simulink model "ANS_GFM_short_term"  (R2021b)
settings: Solver=FixedStepAuto  StartTime=0.0  StopTime=5  FixedStep=Ts  MaxStep=1e-5  RelTol=1e-3
values from neighbouring files (symbols this model uses):
  angle_load = angle(LF.bus(ind_l).Vbus)*180/pi    [init_ANS_GFM_long_term.m]    (also in init_ANS_GFM_short_term.m)
  angleV_LF = Vangle_init/180*pi    [init_ANS_GFM_long_term.m]    (also in init_ANS_GFM_short_term.m)
  awu = 1    [init_ANS_GFM_long_term.m]    (also in init_ANS_GFM_short_term.m)
  C_dc = 1/(Xcdc_pu_or*Zbase_dc_new*100*pi)    [init_ANS_GFM_long_term.m]    (also in init_ANS_GFM_short_term.m)
  C_f = 1/(Xcf_pu_or*Zbase_new*100*pi)    (= 0.013712)    [init_ANS_GFM_long_term.m]    (also in init_ANS_GFM_short_term.m = 0.0141333333333)
  control = 3    [init_ANS_GFM_long_term.m]    (also in init_ANS_GFM_short_term.m = 1)
  D_p = (1/(m_p*w_b))    (= 5209935.26289)    [init_ANS_GFM_long_term.m]    (also in init_ANS_GFM_short_term.m = 5370022.73304)
  Egrid_tmp = 1.054080675694902*400e3    (= 421632.270278)    [init_ANS_GFM_long_term.m]    (also in init_ANS_GFM_short_term.m)
  epsi = 1e-4    (= 0.0001)    [init_ANS_GFM_long_term.m]    (also in init_ANS_GFM_short_term.m)
  eta = m_p*V_m^2    [init_ANS_GFM_long_term.m]    (also in init_ANS_GFM_short_term.m)
  gamma = 2.3    [init_ANS_GFM_long_term.m]    (also in init_ANS_GFM_short_term.m)
  I0_init = [I0_init_a, I0_init_b, I0_init_c]    [init_ANS_GFM_long_term.m]    (also in init_ANS_GFM_short_term.m)
  I_bc = S_bc / (V_bc*sqrt(3))    [init_ANS_GFM_long_term.m]    (also in init_ANS_GFM_short_term.m)
  I_d_int_init = (U_d_int + I_q_int*L_f*w_b - V_d_int - I_d_int*R_f*0)    [init_ANS_GFM_long_term.m]    (also in init_ANS_GFM_short_term.m)
  I_init = [I_init_a, I_init_b, I_init_c]    [init_ANS_GFM_long_term.m]    (also in init_ANS_GFM_short_term.m)
  i_ll = -1.15*(S_bc/Vdc_n)-i_loss_dc    [init_ANS_GFM_long_term.m]    (also in init_ANS_GFM_short_term.m)
  I_max_sat_pu = 1.0 * I_bc *sqrt(2)    [init_ANS_GFM_long_term.m]    (also in init_ANS_GFM_short_term.m)
  I_q_int_init = (U_q_int - I_d_int*L_f*w_b - V_q_int - I_q_int*R_f*0)    [init_ANS_GFM_long_term.m]    (also in init_ANS_GFM_short_term.m)
  i_ul = 1.15*(S_bc/Vdc_n)+i_loss_dc    [init_ANS_GFM_long_term.m]    (also in init_ANS_GFM_short_term.m)
  idppu = 0.95    [init_ANS_GFM_long_term.m]    (also in init_ANS_GFM_short_term.m = 0.92)
  init_dP = -inv(A_pm)*B_pm*dP    [init_ANS_GFM_long_term.m]    (also in init_ANS_GFM_short_term.m)
  init_pm = -inv(A_pm)*B_pm*P_aft    [init_ANS_GFM_long_term.m]    (also in init_ANS_GFM_short_term.m)
  init_tau = -inv(A_tau)*B_tau*idc    [init_ANS_GFM_long_term.m]    (also in init_ANS_GFM_short_term.m)
  J = D_p*tau_f    (= 104198.705258)    [init_ANS_GFM_long_term.m]    (also in init_ANS_GFM_short_term.m = 107400.454661)
  k_dc = eta_1/(Vdc_n*m_p)    [init_ANS_GFM_long_term.m]    (also in init_ANS_GFM_short_term.m)
  K_p = (1/Vdc_n)    [init_ANS_GFM_long_term.m]    (also in init_ANS_GFM_short_term.m)
  K_r = 1/R_dc    [init_ANS_GFM_long_term.m]    (also in init_ANS_GFM_short_term.m)
  Kff_i = 1    [init_ANS_GFM_long_term.m]    (also in init_ANS_GFM_short_term.m)
  Kff_v = 1    [init_ANS_GFM_long_term.m]    (also in init_ANS_GFM_short_term.m)
  Ki_i = (1/n)*1.19    (= 0.0520711785298)    [init_ANS_GFM_long_term.m]    (also in init_ANS_GFM_short_term.m = 0.0505188679245)
  Ki_pll = 4255.3    [init_ANS_GFM_long_term.m]    (also in init_ANS_GFM_short_term.m)
  Ki_v = (n)*1.161022    (= 26.5332227733)    [init_ANS_GFM_long_term.m]    (also in init_ANS_GFM_short_term.m = 27.3485182222)
  ki_v_ac = 2*0.25    (= 0.5)    [init_ANS_GFM_long_term.m]    (also in init_ANS_GFM_short_term.m)
  Kp_i = 0.738891/n    (= 0.032331869895)    [init_ANS_GFM_long_term.m]    (also in init_ANS_GFM_short_term.m = 0.0313680141509)
  Kp_pll = 92    [init_ANS_GFM_long_term.m]    (also in init_ANS_GFM_short_term.m)
  Kp_v = 0.52*n    (= 11.8837333333)    [init_ANS_GFM_long_term.m]    (also in init_ANS_GFM_short_term.m = 12.2488888889)
  kp_v_ac = 0.001    [init_ANS_GFM_long_term.m]    (also in init_ANS_GFM_short_term.m)
  Kpl = 5.0    (= 5)    [init_ANS_GFM_long_term.m]    (also in init_ANS_GFM_short_term.m)
  L1 = cf/sqrt(1+RX^2)*(400e3)^2/Skss/(100*pi)    [init_ANS_GFM_long_term.m]    (also in init_ANS_GFM_short_term.m)
  L_f = Xlf_pu_or*Zbase_new/100/pi    (= 4.37572928821e-06)    [init_ANS_GFM_long_term.m]    (also in init_ANS_GFM_short_term.m = 4.24528301887e-06)
  Lf = 1e6/100/pi    (= 3183.09886184)    [init_ANS_GFM_long_term.m]    (also in init_ANS_GFM_short_term.m = 0.0636619772368)
  m_p = (2*pi*0.5)/(S_bc)    (= 6.10967066042e-10)    [init_ANS_GFM_long_term.m]    (also in init_ANS_GFM_short_term.m = 5.92753330866e-10)
  n = 1/Zb    (= 22.8533333333)    [init_ANS_GFM_long_term.m]    (also in init_ANS_GFM_short_term.m = 23.5555555556)
  P_LF_si = P_LF*S_b    [init_ANS_GFM_long_term.m]    (also in init_ANS_GFM_short_term.m)
  ps = 4440e6/S_bc    (= 0.863477246208)    [init_ANS_GFM_long_term.m]    (also in init_ANS_GFM_short_term.m = 0.837735849057)
  Q_LF_si = Q_LF*S_b    [init_ANS_GFM_long_term.m]    (also in init_ANS_GFM_short_term.m)
  qs = Q_LF*S_b/S_bc    [init_ANS_GFM_long_term.m]    (also in init_ANS_GFM_short_term.m)
  R1 = RX*cf/sqrt(1+RX^2)*(400e3)^2/Skss    [init_ANS_GFM_long_term.m]    (also in init_ANS_GFM_short_term.m)
  R_dc = Rdc_pu_or*Zbase_dc_new    [init_ANS_GFM_long_term.m]    (also in init_ANS_GFM_short_term.m)
  R_f = Rf_pu_or*Zbase_new    (= 2.18786464411e-05)    [init_ANS_GFM_long_term.m]    (also in init_ANS_GFM_short_term.m = 2.12264150943e-05)
  Rf = 1e6    (= 1000000)    [init_ANS_GFM_long_term.m]    (also in init_ANS_GFM_short_term.m = 20)
  S_bc = 5142e6    (= 5142000000)    [init_ANS_GFM_long_term.m]    (also in init_ANS_GFM_short_term.m = 5300000000)
  sat_select = 3    [init_ANS_GFM_long_term.m]    (also in init_ANS_GFM_short_term.m)
  SECM = 3    [init_ANS_GFM_long_term.m]    (also in init_ANS_GFM_short_term.m = 1)
  share_i_load = 1.0    (= 1)    [init_ANS_GFM_long_term.m]    (also in init_ANS_GFM_short_term.m)
  T_en = -0.5    [init_ANS_GFM_long_term.m]    (also in init_ANS_GFM_short_term.m)
  T_off = T_on + 0.1    (= 0.2)    [init_ANS_GFM_long_term.m]    (also in init_ANS_GFM_short_term.m)
  T_on = 0.1    [init_ANS_GFM_long_term.m]    (also in init_ANS_GFM_short_term.m)
  Ts = 2e-6    (= 2e-06)    [init_ANS_GFM_long_term.m]    (also in init_ANS_GFM_short_term.m = 1e-06)
  U_init = [Umag_init_a, Umag_init_b, Umag_init_c]    [init_ANS_GFM_long_term.m]    (also in init_ANS_GFM_short_term.m)
  Uangle_init = angle(V_LF_VSC)*180/pi    [init_ANS_GFM_long_term.m]    (also in init_ANS_GFM_short_term.m)
  Umag_init = abs(V_LF_VSC)*V_bc*sqrt(2/3)    [init_ANS_GFM_long_term.m]    (also in init_ANS_GFM_short_term.m)
  V1_rms = 15e3    (= 15000)    [init_ANS_GFM_long_term.m]    (also in init_ANS_GFM_short_term.m)
  V_d_int = abs(V_LF)*V_bc*sqrt(2/3)    [init_ANS_GFM_long_term.m]    (also in init_ANS_GFM_short_term.m)
  V_d_int_init = (I_d_int + V_q_int*C_f*w_b - I0_d_int)    [init_ANS_GFM_long_term.m]    (also in init_ANS_GFM_short_term.m)
  V_init = [V_init_a, V_init_b, V_init_c]    [init_ANS_GFM_long_term.m]    (also in init_ANS_GFM_short_term.m)
  V_m = sqrt(2/3)*V_bc    [init_ANS_GFM_long_term.m]    (also in init_ANS_GFM_short_term.m)
  V_q_int_init = (I_q_int - V_d_int*C_f*w_b - I0_q_int)    [init_ANS_GFM_long_term.m]    (also in init_ANS_GFM_short_term.m)
  Vdc_n = 3*V_m    [init_ANS_GFM_long_term.m]    (also in init_ANS_GFM_short_term.m)
  Vref = V_LF_mag*V_m    [init_ANS_GFM_long_term.m]    (also in init_ANS_GFM_short_term.m)
  w_b = 2*pi*f_b    (= 314.159265359)    [init_ANS_GFM_long_term.m]    (also in init_ANS_GFM_short_term.m)
  w_f = 2*pi*5    (= 31.4159265359)    [init_ANS_GFM_long_term.m]    (also in init_ANS_GFM_short_term.m)
  Zbase_new = V1_rms^2/S_bc    (= 0.0437572928821)    [init_ANS_GFM_long_term.m]    (also in init_ANS_GFM_short_term.m = 0.0424528301887)
undefined symbols (not defined in the file or in its folder): A_pm, A_tau, B_pm, B_tau, C_pm, C_tau, D_pm, D_tau, find_system, idq0_init, Pm, sm_init, v_d, v_q, Ve
libraries: spsBreakerLib x270, spsGroundLib x21, spsThreePhaseSeriesRLCBranchLib x12, spsabctodq0Lib x11, simulink x9, spsEdgeDetectorLib x8, spsThreePhaseVIMeasurementLib x7, spsLoadFlowBusLib x7, spsSeriesRLCBranchLib x6, spsControlledVoltageSourceLib x6, spsCurrentMeasurementLib x6, spsVoltageMeasurementLib x6
(part 3 of 7)

== system ANS_GFM_short_term/GFM Converter/Current Loop1 ==
  i_s_ref_dq0 : Inport
  v_dq0 : Inport  Port=2
  i_s_dq0 : Inport  Port=3
  w : Inport  Port=4
  Demux : Demux  Outputs=2
  Demux1 : Demux  Outputs=2
  Demux2 : Demux  Outputs=2
  Gain Corrector : Gain  Commented=through  Gain=Kp_i
  Gain Corrector1 : Gain  Commented=through  Gain=Kp_i
  Gain Corrector2 : Gain  Gain=Kp_i
  Gain Corrector3 : Gain  Gain=Kp_i
  Integration Time : Gain  Gain=Ki_i
  Integration Time 1 : Gain  Gain=Ki_i
  Integration Time1 : Gain  Commented=on  Gain=1/n
  Integration Time2 : Gain  Commented=on  Gain=1/n
  Integrator : Integrator  InitialCondition=I_d_int_init
  Integrator 1 : Integrator  InitialCondition=I_q_int_init
  Mux : Mux  Inputs=3
  Product : Product  RndMeth=Zero
  Product1 : Product  RndMeth=Zero
  Selector1 : Selector  InputPortWidth=3  IndexOptions=Index vector (dialog)  Indices=[1 2]  OutputSizes=1
  Selector2 : Selector  InputPortWidth=3  IndexOptions=Index vector (dialog)  Indices=[1 2]  OutputSizes=1
  Selector3 : Selector  InputPortWidth=3  IndexOptions=Index vector (dialog)  Indices=[1 2]  OutputSizes=1
  Sum : Sum  Inputs=|+-
  Sum1 : Sum  Inputs=|++
  Sum2 : Sum  Inputs=|+-
  Sum3 : Sum  Inputs=|++
  Sum4 : Sum  Inputs=|++
  Sum5 : Sum  Inputs=++|
  Sum6 : Sum  Inputs=-+|
  Sum7 : Sum  Inputs=++|
  Vm_0* : Constant  Value=0
  Voltage Compensator 1 : Gain  Gain=Kff_v
  Voltage compensator : Gain  Gain=Kff_v
  w*Lf_pu : Gain  Gain=L_f
  v_s_ref_dq0 : Outport  VectorParamsAs1DForOutWhenUnconnected=off
  wires:
  Gain Corrector1/1 -> Sum5/2
  Product1/1 -> Sum5/1
  Demux2/1 -> Voltage compensator/1
  Demux1/1 -> Sum/2, Product1/2
  Integrator/1 -> Sum1/1
  Vm_0*/1 -> Mux/3
  Demux1/2 -> Sum6/1, Product/1
  Selector3/1 -> Demux2/1
  i_s_dq0/1 -> Selector2/1
  Selector2/1 -> Demux1/1
  Mux/1 -> v_s_ref_dq0/1
  w/1 -> w*Lf_pu/1
  Gain Corrector/1 -> Sum2/1
  Selector1/1 -> Demux/1
  Demux/2 -> Sum6/2
  Sum4/1 -> Gain Corrector1/1
  Sum2/1 -> Sum3/1
  Sum1/1 -> Gain Corrector/1
  Voltage compensator/1 -> Sum3/2
  Integrator 1/1 -> Sum4/1
  v_dq0/1 -> Selector3/1
  i_s_ref_dq0/1 -> Selector1/1
  w*Lf_pu/1 -> Product/2, Product1/1
  Product/1 -> Sum2/2
  Voltage Compensator 1/1 -> Sum7/1
  Demux2/2 -> Voltage Compensator 1/1
  Sum7/1 -> Mux/2  "Vm_q*"
  Sum3/1 -> Mux/1  "Vm_d*"
  Demux/1 -> Sum/1
  Sum6/1 -> Integration Time 1/1, Gain Corrector3/1
  Sum5/1 -> Sum7/2
  Integration Time/1 -> Integrator/1
  Integration Time 1/1 -> Integrator 1/1
  Sum/1 -> Integration Time/1, Gain Corrector2/1
  Gain Corrector2/1 -> Sum1/2
  Gain Corrector3/1 -> Sum4/2

== system ANS_GFM_short_term/GFM Converter/GFM controls ==
  chosen_control : Inport
  P_abc : Inport  Port=2
  P_set : Inport  Port=3
  v_abc : Inport  Port=4
  v_dc : Inport  Port=5
  Q_abc : Inport  Port=6
  dv_q : Inport  Port=7
  Q_set : Inport  Port=8
  anti-windup : Inport  Port=9
  Compare To Constant1 : simulink/Logic and Bit Operations/Compare To Constant  relop===  const=1  OutDataTypeStr=boolean
  Compare To Constant2 : simulink/Logic and Bit Operations/Compare To Constant  relop===  const=2  OutDataTypeStr=boolean
  Compare To Constant3 : simulink/Logic and Bit Operations/Compare To Constant  relop===  const=3  OutDataTypeStr=boolean
  Compare To Constant4 : simulink/Logic and Bit Operations/Compare To Constant  relop===  const=4  OutDataTypeStr=boolean
  Constant : Constant  Value=w_b
  Constant1 : Constant  Value=Vref
  Demux : Demux  Outputs=3
  Droop Control : Subsystem
  Matching Control : Subsystem
  Multiport Switch : MultiPortSwitch  Inputs=4
  Mux{,1..3} (4 alike) : Mux  Inputs=3
  VSM Control : Subsystem
  dVOC  - kappa=pi/2 : Subsystem
  w_ref : Outport
  theta_ref : Outport  Port=2
  v_ref_dqo : Outport  Port=3
  wires:
  Droop Control/1(w_ref) -> Mux/1
  Droop Control/2(theta_ref) -> Mux/2
  Droop Control/3(v_ref_dq0) -> Mux/3
  Compare To Constant1/1 -> Droop Control/Enable
  Compare To Constant2/1 -> Matching Control/Enable
  Compare To Constant3/1 -> dVOC  - kappa=pi/2/Enable
  Compare To Constant4/1 -> VSM Control/Enable
  Constant/1 -> Droop Control/1(w_b), VSM Control/5(w_b), dVOC  - kappa=pi/2/1(w_b)
  Constant1/1 -> VSM Control/3(v_m), dVOC  - kappa=pi/2/4(v_m), Matching Control/3(v_m), Droop Control/4(v_m)
  Matching Control/1(w_ref) -> Mux1/1
  Matching Control/3(v_ref_dq0) -> Mux1/3
  Matching Control/2(theta_ref) -> Mux1/2
  dVOC  - kappa=pi/2/1(w_ref) -> Mux2/1
  dVOC  - kappa=pi/2/3(v_ref_dq0) -> Mux2/3
  dVOC  - kappa=pi/2/2(theta_ref) -> Mux2/2
  VSM Control/1(w_ref) -> Mux3/1
  VSM Control/3(v_ref_dq0) -> Mux3/3
  VSM Control/2(theta_ref) -> Mux3/2
  Multiport Switch/1 -> Demux/1
  Demux/1 -> w_ref/1
  Demux/2 -> theta_ref/1
  Demux/3 -> v_ref_dqo/1
  Mux3/1 -> Multiport Switch/5
  Mux2/1 -> Multiport Switch/4
  Mux1/1 -> Multiport Switch/3
  Mux/1 -> Multiport Switch/2
  P_abc/1 -> VSM Control/1(p_m), dVOC  - kappa=pi/2/2(p_m), Droop Control/2(p_m)
  v_abc/1 -> Matching Control/2(V_abc), Droop Control/5(V_abc), VSM Control/4(V_abc)
  v_dc/1 -> Matching Control/1(v_dc)
  Q_abc/1 -> dVOC  - kappa=pi/2/5(q_m)
  P_set/1 -> Droop Control/3(p_set), VSM Control/2(p_set), dVOC  - kappa=pi/2/3(p_set)
  anti-windup/1 -> Droop Control/6(anti-windup), Matching Control/4(anti-windup), dVOC  - kappa=pi/2/7(anti-windup), VSM Control/6(anti-windup)
  Q_set/1 -> dVOC  - kappa=pi/2/6(q_set)
  chosen_control/1 -> Compare To Constant4/1, Compare To Constant3/1, Compare To Constant2/1, Multiport Switch/1, Compare To Constant1/1
  dv_q/1 -> VSM Control/7(dv_q), dVOC  - kappa=pi/2/8(dv_q), Matching Control/5(dv_q), Droop Control/7(dv_q)

== system ANS_GFM_short_term/GFM Converter/PT1 ==
  in : Inport
  Gain15 : Gain  Gain=1/1e-4
  Integrator : Integrator  InitialCondition=ps*S_bc
  Sum6 : Sum  Inputs=|+-
  out : Outport
  wires:
  Integrator/1 -> out/1, Sum6/2
  Gain15/1 -> Integrator/1
  Sum6/1 -> Gain15/1
  in/1 -> Sum6/1

== system ANS_GFM_short_term/GFM Converter/PT2 ==
  in : Inport
  Gain15 : Gain  Gain=1/1e-4
  Integrator : Integrator
  Sum6 : Sum  Inputs=|+-
  out : Outport
  wires:
  Integrator/1 -> out/1, Sum6/2
  Gain15/1 -> Integrator/1
  Sum6/1 -> Gain15/1
  in/1 -> Sum6/1

== system ANS_GFM_short_term/GFM Converter/PT3 ==
  in : Inport
  Gain15 : Gain  Gain=1/1e-4
  Integrator : Integrator  InitialCondition=qs*S_bc
  Sum6 : Sum  Inputs=|+-
  out : Outport
  wires:
  Integrator/1 -> out/1, Sum6/2
  Gain15/1 -> Integrator/1
  Sum6/1 -> Gain15/1
  in/1 -> Sum6/1

== system ANS_GFM_short_term/GFM Converter/SECMs ==
  secm : Inport
  pset : Inport  Port=2
  imax_flag : Inport  Port=3
  V_dq0 : Inport  Port=4
  i_dqlim : Inport  Port=5
  i_s_dq0 : Inport  Port=6
  qset0 : Inport  Port=7
  Compare To Constant1 : simulink/Logic and Bit Operations/Compare To Constant  relop===  const=1  OutDataTypeStr=boolean
  Compare To Constant2 : simulink/Logic and Bit Operations/Compare To Constant  relop===  const=2  OutDataTypeStr=boolean
  Compare To Constant3 : simulink/Logic and Bit Operations/Compare To Constant  relop===  const=3  OutDataTypeStr=boolean
  Compare To Constant4 : simulink/Logic and Bit Operations/Compare To Constant  relop===  const=4  OutDataTypeStr=boolean
  Demux : Demux  Outputs=3
  Gain : Gain  Gain=1/V_m
  Gain1 : Gain  Gain=1/V_m
  Multiport Switch : MultiPortSwitch  Inputs=5
  Multiport Switch1 : MultiPortSwitch  Inputs=5
  SECM-1 : Subsystem
  SECM-2 : Subsystem
  SECM-3 : Subsystem
  SECM-4 : Subsystem
  Square : Math  Operator=square  SaturateOnIntegerOverflow=on
  Square Root : Sqrt  SaturateOnIntegerOverflow=on
  Sum of Elements : Sum  Inputs=+
  pset* : Outport
  dv_q : Outport  Port=2
  qset* : Outport  Port=3
  wires:
  secm/1 -> Compare To Constant3/1, Compare To Constant4/1, Compare To Constant2/1, Compare To Constant1/1, Multiport Switch1/1, Multiport Switch/1
  Multiport Switch/1 -> pset*/1
  Square/1 -> Sum of Elements/1
  Sum of Elements/1 -> Square Root/1
  Square Root/1 -> Gain/1
  Demux/2 -> Gain1/1
  SECM-3/2(dv_q) -> dv_q/1
  V_dq0/1 -> SECM-1/3(Vdq0), Square/1, Demux/1
  Multiport Switch1/1 -> qset*/1
  Compare To Constant1/1 -> SECM-1/Enable
  Compare To Constant2/1 -> SECM-2/Enable
  Compare To Constant3/1 -> SECM-3/Enable
  Compare To Constant4/1 -> SECM-4/Enable
  SECM-4/1(pset*) -> Multiport Switch/5
  SECM-3/1(pset*) -> Multiport Switch/4
  SECM-2/1(pset*) -> Multiport Switch/3
  SECM-1/1(pset*) -> Multiport Switch/2
  SECM-1/2(qset*) -> Multiport Switch1/2
  qset0/1 -> SECM-1/5(Qset0), Multiport Switch1/4, Multiport Switch1/5, Multiport Switch1/6, Multiport Switch1/3
  imax_flag/1 -> SECM-1/2(imax_flag)
  i_dqlim/1 -> SECM-1/4(Idq0_lim)
  pset/1 -> SECM-4/1(pset), Multiport Switch/6, SECM-3/1(pset), SECM-2/1(pset), SECM-1/1(Pset0)
  Gain1/1 -> SECM-3/2(V_q_pu)
  i_s_dq0/1 -> SECM-4/2(i_s_dq0)
  Gain/1 -> SECM-2/2(V_pu)

== system ANS_GFM_short_term/GFM Converter/Voltage Loop1 ==
  v_ref_dq0 : Inport
  v_dq0 : Inport  Port=2
  i_dq0 : Inport  Port=3
  w : Inport  Port=4
  anti-windup : Inport  Port=5
  Constant : Constant  Value=0
  Constant1 : Constant  Value=0
  Current Compensator : Gain  Gain=Kff_i
  Current Compensator1 : Gain  Gain=Kff_i
  Damping (d) : Gain  Commented=through  Gain=Kp_v
  Damping (q) : Gain  Commented=through  Gain=Kp_v
  Demux : Demux  Outputs=2
  Demux1 : Demux  Outputs=2
  Demux2 : Demux  Outputs=2
  Eg_d * (wCf) : Product  RndMeth=Zero
  "Eg_q * (wCf) " : Product  RndMeth=Zero
  Filter capacitance : Gain  Gain=C_f
  Integration Time : Gain  Gain=Ki_v
  Integration Time1 : Gain  Gain=Ki_v
  Integration Time2 : Gain  Gain=Kp_v
  Integration Time3 : Gain  Gain=Kp_v
  Integrator : Integrator  InitialCondition=V_d_int_init
  Integrator1 : Integrator  InitialCondition=V_q_int_init
  Is_0* : Constant  Value=0
  Mux : Mux  Inputs=3
  Selector : Selector  InputPortWidth=3  IndexOptions=Index vector (dialog)  Indices=[1 2]  OutputSizes=1
  Selector1 : Selector  InputPortWidth=3  IndexOptions=Index vector (dialog)  Indices=[1 2]  OutputSizes=1
  Selector2 : Selector  InputPortWidth=3  IndexOptions=Index vector (dialog)  Indices=[1 2]  OutputSizes=1
  Sum : Sum  Inputs=|+-
  Sum1 : Sum  Inputs=|++
  Sum2 : Sum  Inputs=|+-
  Sum3 : Sum  Inputs=|++
  Sum4 : Sum  Inputs=|++
  Sum5 : Sum  Inputs=++|
  Sum6 : Sum  Inputs=-+|
  Sum7 : Sum  Inputs=++|
  Switch1 : Switch  Criteria=u2 > Threshold
  Switch2 : Switch  Criteria=u2 > Threshold
  i_s_ref_dq0 : Outport  VectorParamsAs1DForOutWhenUnconnected=off
  wires:
  Integration Time3/1 -> Sum4/2
  Integration Time2/1 -> Sum1/2
  Sum/1 -> Integration Time2/1, Integration Time/1
  Mux/1 -> i_s_ref_dq0/1
  Selector2/1 -> Demux2/1
  Selector1/1 -> Demux/1
  Selector/1 -> Demux1/1
  Damping (q)/1 -> Sum5/2  "Is_q\""
  v_dq0/1 -> Selector/1
  Sum3/1 -> Mux/1  "Is_d*"
  Sum4/1 -> Damping (q)/1
  Integrator/1 -> Sum1/1
  Sum1/1 -> Damping (d)/1
  Sum5/1 -> Sum7/2  "Is_q'"
  i_dq0/1 -> Selector2/1
  Damping (d)/1 -> Sum2/1  "Is_d\""
  Filter capacitance/1 -> Eg_d * (wCf)/2, "Eg_q * (wCf) "/2
  Demux1/2 -> Sum6/1, "Eg_q * (wCf) "/1  "Eg_q"
  "Eg_q * (wCf) "/1 -> Sum2/2  "Is_f"
  Current Compensator1/1 -> Sum7/1
  Demux1/1 -> Sum/2, Eg_d * (wCf)/1  "Eg_d"
  Current Compensator/1 -> Sum3/2
  Sum2/1 -> Sum3/1  "Is_d'"
  Demux2/1 -> Current Compensator/1  "Ig_d"
  Sum6/1 -> Integration Time3/1, Integration Time1/1
  Demux/1 -> Sum/1  "Eg_d*"
  Demux2/2 -> Current Compensator1/1  "Ig_q"
  Sum7/1 -> Mux/2  "Is_q*"
  Eg_d * (wCf)/1 -> Sum5/1  "Is_f"
  v_ref_dq0/1 -> Selector1/1
  Demux/2 -> Sum6/2  "Eg_q*"
  Integrator1/1 -> Sum4/1
  w/1 -> Filter capacitance/1
  Is_0*/1 -> Mux/3
  Switch2/1 -> Integrator/1
  Integration Time/1 -> Switch2/1
  anti-windup/1 -> Switch1/2, Switch2/2
  Constant/1 -> Switch2/3
  Switch1/1 -> Integrator1/1
  Constant1/1 -> Switch1/3
  Integration Time1/1 -> Switch1/1

== system ANS_GFM_short_term/OLTC/ OLTC Control ==
  note: The 2 resistors are in operation during TransferTime/3
  note: Tap changer Mechanical Delay= TapSelectionTime
  Up : Inport
  Down : Inport  Port=2
  Abs1 : Abs  SaturateOnIntegerOverflow=on
  Constant : Constant  Value=TapVector
  Edge Detector : spsEdgeDetectorLib/Edge Detector  model=Rising  ic=0  Ts=0
      settings: SourceProductBaseCode=PS
  Logical Operator : Logic  Operator=NOT  AllPortsSameDT=off
  Monostable1 : spsMonostableLib/Monostable  EdgeDetect=Rising  PulseDuration=TransferTime  ic=1  Ts=0
      settings: SourceProductBaseCode=PS
  Off Delay : spsOnDelayLib/On Delay  DelayType=Off delay  delay=2*TransferTime/3  ic=InitialStates  Ts=0
      settings: SourceProductBaseCode=PS
  On Delay : spsOnDelayLib/On Delay  DelayType=On delay  delay=TransferTime/3  ic=1  Ts=0
      settings: SourceProductBaseCode=PS
  Relational Operator : RelationalOperator  Operator===  RndMeth=Nearest
  S-R Flip-Flop : simulink_extras/Flip Flops/S-R Flip-Flop  initial_condition=InitialTap>=0
  Set Reset : Subsystem
  Tap Changer Control : Subsystem  mask(Tap Changer Control){MinMaxTap=[-NumberOfTaps  +NumberOfTaps], InitialPosition=InitialTap, MecDelay=TapSelectionTime}
      mask prompts: MinMaxTap "Minimum and maximum tap number [ Min  Max ] :"; InitialPosition "Initial tap position"; MecDelay "Mechanical delay time"
      mask init:
      | if MecDelay<=0,
      | 	MecDelay=1/60;
      | end
  Terminator1 : Terminator
  Tap : Outport  VectorParamsAs1DForOutWhenUnconnected=off
  SwSelect : Outport  Port=2  VectorParamsAs1DForOutWhenUnconnected=off
  SwTr : Outport  Port=3  VectorParamsAs1DForOutWhenUnconnected=off
  SwInv : Outport  Port=4  VectorParamsAs1DForOutWhenUnconnected=off
  Ready : Outport  Port=5  VectorParamsAs1DForOutWhenUnconnected=off
  wires:
  Constant/1 -> Relational Operator/2
  Logical Operator/1 -> SwTr/1
  Down/1 -> Tap Changer Control/2(Down)
  Up/1 -> Tap Changer Control/1(Up)
  Relational Operator/1 -> On Delay/1
  Monostable1/1 -> Logical Operator/1
  Tap Changer Control/1(TapNo) -> Tap/1, Edge Detector/1, Set Reset/1(Tap), Abs1/1
  Tap Changer Control/2(Ready) -> Ready/1
  S-R Flip-Flop/2 -> Terminator1/1
  Edge Detector/1 -> Monostable1/1
  S-R Flip-Flop/1 -> SwInv/1
  Abs1/1 -> Relational Operator/1
  On Delay/1 -> Off Delay/1
  Off Delay/1 -> SwSelect/1
  Set Reset/1(Set) -> S-R Flip-Flop/1
  Set Reset/2(Reset) -> S-R Flip-Flop/2

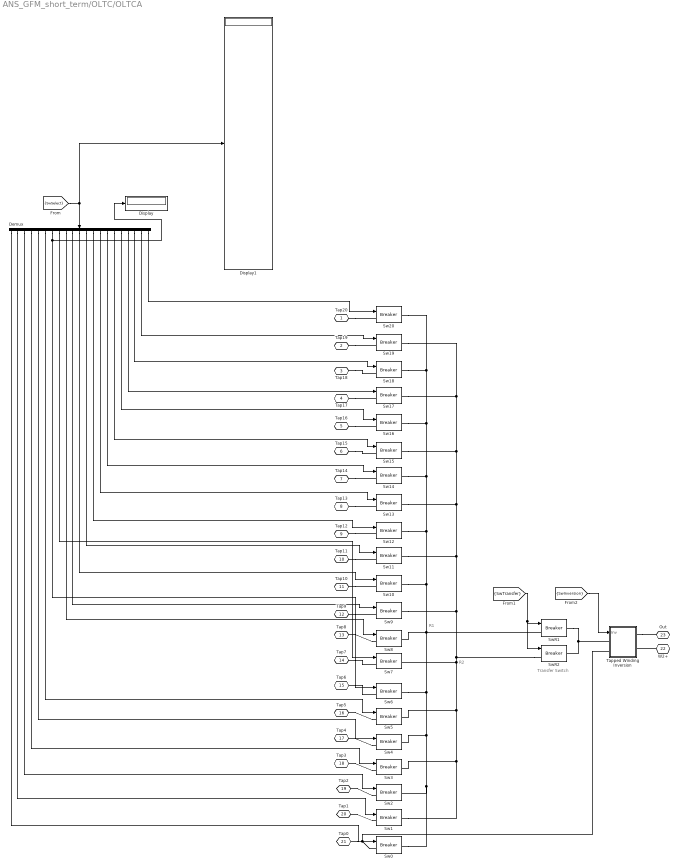
== system ANS_GFM_short_term/OLTC/OLTCA ==
  note: R2
  note: R1
  note: Transfer Switch
  Demux : Demux  Outputs=21
      settings: DisplayOption=none
  Display : Display
  Display1 : Display
  "Sw0 " : spsBreakerLib/Breaker  InitialState=InitialStates(1)  SwitchingTimes="[ 1/60  5/60 ]"  External=on  BreakerResistance=Rswitch  SnubberResistance=1e8  SnubberCapacitance=inf  Measurements=None  MoreParameters=off  NoBreakLoop=off
      settings: SourceProductBaseCode=PS
  "Sw1 " : spsBreakerLib/Breaker  InitialState=InitialStates(2)  SwitchingTimes="[ 1/60  5/60 ]"  External=on  BreakerResistance=Rswitch  SnubberResistance=1e8  SnubberCapacitance=inf  Measurements=None  MoreParameters=off  NoBreakLoop=off
      settings: SourceProductBaseCode=PS
  Sw10 : spsBreakerLib/Breaker  InitialState=InitialStates(11)  SwitchingTimes="[ 1/60  5/60 ]"  External=on  BreakerResistance=Rswitch  SnubberResistance=1e8  SnubberCapacitance=inf  Measurements=None  MoreParameters=off  NoBreakLoop=off
      settings: SourceProductBaseCode=PS
  Sw11 : spsBreakerLib/Breaker  InitialState=InitialStates(12)  SwitchingTimes="[ 1/60  5/60 ]"  External=on  BreakerResistance=Rswitch  SnubberResistance=1e8  SnubberCapacitance=inf  Measurements=None  MoreParameters=off  NoBreakLoop=off
      settings: SourceProductBaseCode=PS
  Sw12 : spsBreakerLib/Breaker  InitialState=InitialStates(13)  SwitchingTimes="[ 1/60  5/60 ]"  External=on  BreakerResistance=Rswitch  SnubberResistance=1e8  SnubberCapacitance=inf  Measurements=None  MoreParameters=off  NoBreakLoop=off
      settings: SourceProductBaseCode=PS
  Sw13 : spsBreakerLib/Breaker  InitialState=InitialStates(14)  SwitchingTimes="[ 1/60  5/60 ]"  External=on  BreakerResistance=Rswitch  SnubberResistance=1e8  SnubberCapacitance=inf  Measurements=None  MoreParameters=off  NoBreakLoop=off
      settings: SourceProductBaseCode=PS
  Sw14 : spsBreakerLib/Breaker  InitialState=InitialStates(15)  SwitchingTimes="[ 1/60  5/60 ]"  External=on  BreakerResistance=Rswitch  SnubberResistance=1e8  SnubberCapacitance=inf  Measurements=None  MoreParameters=off  NoBreakLoop=off
      settings: SourceProductBaseCode=PS
  Sw15 : spsBreakerLib/Breaker  InitialState=InitialStates(16)  SwitchingTimes="[ 1/60  5/60 ]"  External=on  BreakerResistance=Rswitch  SnubberResistance=1e8  SnubberCapacitance=inf  Measurements=None  MoreParameters=off  NoBreakLoop=off
      settings: SourceProductBaseCode=PS
  Sw16 : spsBreakerLib/Breaker  InitialState=InitialStates(17)  SwitchingTimes="[ 1/60  5/60 ]"  External=on  BreakerResistance=Rswitch  SnubberResistance=1e8  SnubberCapacitance=inf  Measurements=None  MoreParameters=off  NoBreakLoop=off
      settings: SourceProductBaseCode=PS
  Sw17 : spsBreakerLib/Breaker  InitialState=InitialStates(18)  SwitchingTimes="[ 1/60  5/60 ]"  External=on  BreakerResistance=Rswitch  SnubberResistance=1e8  SnubberCapacitance=inf  Measurements=None  MoreParameters=off  NoBreakLoop=off
      settings: SourceProductBaseCode=PS
  Sw18 : spsBreakerLib/Breaker  InitialState=InitialStates(19)  SwitchingTimes="[ 1/60  5/60 ]"  External=on  BreakerResistance=Rswitch  SnubberResistance=1e8  SnubberCapacitance=inf  Measurements=None  MoreParameters=off  NoBreakLoop=off
      settings: SourceProductBaseCode=PS
  Sw19 : spsBreakerLib/Breaker  InitialState=InitialStates(20)  SwitchingTimes="[ 1/60  5/60 ]"  External=on  BreakerResistance=Rswitch  SnubberResistance=1e8  SnubberCapacitance=inf  Measurements=None  MoreParameters=off  NoBreakLoop=off
      settings: SourceProductBaseCode=PS
  "Sw2 " : spsBreakerLib/Breaker  InitialState=InitialStates(3)  SwitchingTimes="[ 1/60  5/60 ]"  External=on  BreakerResistance=Rswitch  SnubberResistance=1e8  SnubberCapacitance=inf  Measurements=None  MoreParameters=off  NoBreakLoop=off
      settings: SourceProductBaseCode=PS
  Sw20 : spsBreakerLib/Breaker  InitialState=InitialStates(21)  SwitchingTimes="[ 1/60  5/60 ]"  External=on  BreakerResistance=Rswitch  SnubberResistance=Rsnubber  SnubberCapacitance=inf  Measurements=None  MoreParameters=off  NoBreakLoop=off
      settings: SourceProductBaseCode=PS
  "Sw3 " : spsBreakerLib/Breaker  InitialState=InitialStates(4)  SwitchingTimes="[ 1/60  5/60 ]"  External=on  BreakerResistance=Rswitch  SnubberResistance=1e8  SnubberCapacitance=inf  Measurements=None  MoreParameters=off  NoBreakLoop=off
      settings: SourceProductBaseCode=PS
  "Sw4 " : spsBreakerLib/Breaker  InitialState=InitialStates(5)  SwitchingTimes="[ 1/60  5/60 ]"  External=on  BreakerResistance=Rswitch  SnubberResistance=1e8  SnubberCapacitance=inf  Measurements=None  MoreParameters=off  NoBreakLoop=off
      settings: SourceProductBaseCode=PS
  "Sw5 " : spsBreakerLib/Breaker  InitialState=InitialStates(6)  SwitchingTimes="[ 1/60  5/60 ]"  External=on  BreakerResistance=Rswitch  SnubberResistance=1e8  SnubberCapacitance=inf  Measurements=None  MoreParameters=off  NoBreakLoop=off
      settings: SourceProductBaseCode=PS
  "Sw6 " : spsBreakerLib/Breaker  InitialState=InitialStates(7)  SwitchingTimes="[ 1/60  5/60 ]"  External=on  BreakerResistance=Rswitch  SnubberResistance=1e8  SnubberCapacitance=inf  Measurements=None  MoreParameters=off  NoBreakLoop=off
      settings: SourceProductBaseCode=PS
  "Sw7 " : spsBreakerLib/Breaker  InitialState=InitialStates(8)  SwitchingTimes="[ 1/60  5/60 ]"  External=on  BreakerResistance=Rswitch  SnubberResistance=1e8  SnubberCapacitance=inf  Measurements=None  MoreParameters=off  NoBreakLoop=off
      settings: SourceProductBaseCode=PS
  "Sw8 " : spsBreakerLib/Breaker  InitialState=InitialStates(9)  SwitchingTimes="[ 1/60  5/60 ]"  External=on  BreakerResistance=Rswitch  SnubberResistance=1e8  SnubberCapacitance=inf  Measurements=None  MoreParameters=off  NoBreakLoop=off
      settings: SourceProductBaseCode=PS
  Sw9 : spsBreakerLib/Breaker  InitialState=InitialStates(10)  SwitchingTimes="[ 1/60  5/60 ]"  External=on  BreakerResistance=Rswitch  SnubberResistance=1e8  SnubberCapacitance=inf  Measurements=None  MoreParameters=off  NoBreakLoop=off
      settings: SourceProductBaseCode=PS
  SwR1 : spsBreakerLib/Breaker  InitialState=1  SwitchingTimes="[ 1/60  5/60 ]"  External=on  BreakerResistance=Rswitch  SnubberResistance=Rtransfer  SnubberCapacitance=inf  Measurements=None  MoreParameters=off  NoBreakLoop=off
      settings: SourceProductBaseCode=PS
  SwR2 : spsBreakerLib/Breaker  InitialState=1  SwitchingTimes="[ 1/60  5/60 ]"  External=on  BreakerResistance=Rswitch  SnubberResistance=Rtransfer  SnubberCapacitance=inf  Measurements=None  MoreParameters=off  NoBreakLoop=off
      settings: SourceProductBaseCode=PS
  Tapped Winding Inversion : Subsystem
  Tap20 : PMIOPort  Side=Right
  Tap19 : PMIOPort  Port=2  Side=Right
  Tap18 : PMIOPort  Port=3  Side=Right
  Tap17 : PMIOPort  Port=4  Side=Right
  Tap16 : PMIOPort  Port=5  Side=Right
  Tap15 : PMIOPort  Port=6  Side=Right
  Tap14 : PMIOPort  Port=7  Side=Right
  Tap13 : PMIOPort  Port=8  Side=Right
  Tap12 : PMIOPort  Port=9  Side=Right
  Tap11 : PMIOPort  Port=10  Side=Right
  Tap10 : PMIOPort  Port=11  Side=Right
  Tap9 : PMIOPort  Port=12  Side=Right
  Tap8 : PMIOPort  Port=13  Side=Right
  Tap7 : PMIOPort  Port=14  Side=Right
  Tap6 : PMIOPort  Port=15  Side=Right
  Tap5 : PMIOPort  Port=16  Side=Right
  Tap4 : PMIOPort  Port=17  Side=Right
  Tap3 : PMIOPort  Port=18  Side=Right
  Tap2 : PMIOPort  Port=19  Side=Right
  Tap1 : PMIOPort  Port=20  Side=Right
  Tap0 : PMIOPort  Port=21  Side=Right
  W2+ : PMIOPort  Port=22  Side=Right
  Out : PMIOPort  Port=23  Side=Left
  wires:
  Demux/9 -> "Sw8 "/1
  Demux/8 -> "Sw7 "/1
  Demux/7 -> Display/1, "Sw6 "/1
  Demux/6 -> "Sw5 "/1
  Demux/5 -> "Sw4 "/1
  Demux/4 -> "Sw3 "/1
  Demux/3 -> "Sw2 "/1
  Demux/2 -> "Sw1 "/1
  Demux/1 -> "Sw0 "/1
  [SwInversion] -> Tapped Winding Inversion/1(Inv)
  [SwTransfer] -> SwR2/1, SwR1/1
  [SwSelect] -> Demux/1, Display1/1
  Demux/10 -> Sw9/1
  Demux/11 -> Sw10/1
  Demux/12 -> Sw11/1
  Demux/13 -> Sw12/1
  Demux/14 -> Sw13/1
  Demux/15 -> Sw14/1
  Demux/16 -> Sw15/1
  Demux/17 -> Sw16/1
  Demux/18 -> Sw17/1
  Demux/19 -> Sw18/1
  Demux/20 -> Sw19/1
  Demux/21 -> Sw20/1
  connections:
  "Sw0 "/LConn1 -- Tap0/RConn1 -- Tapped Winding Inversion/LConn2
  Tap1/RConn1 -- "Sw1 "/LConn1
  Tap2/RConn1 -- "Sw2 "/LConn1
  Tap6/RConn1 -- "Sw6 "/LConn1
  Tap4/RConn1 -- "Sw4 "/LConn1
  Tap5/RConn1 -- "Sw5 "/LConn1
  SwR1/RConn1 -- Tapped Winding Inversion/LConn1 -- SwR2/RConn1
  SwR2/LConn1 -- "Sw5 "/RConn1 -- "Sw3 "/RConn1 -- "Sw1 "/RConn1 -- "Sw7 "/RConn1 -- Sw19/RConn1 -- Sw17/RConn1 -- Sw15/RConn1 -- Sw13/RConn1 -- Sw11/RConn1 -- Sw9/RConn1
  Tapped Winding Inversion/RConn1 -- Out/RConn1
  W2+/RConn1 -- Tapped Winding Inversion/RConn2
  "Sw6 "/RConn1 -- Sw20/RConn1 -- Sw18/RConn1 -- Sw16/RConn1 -- Sw14/RConn1 -- Sw12/RConn1 -- Sw10/RConn1 -- "Sw8 "/RConn1 -- SwR1/LConn1 -- "Sw4 "/RConn1 -- "Sw2 "/RConn1 -- "Sw0 "/RConn1
  Tap3/RConn1 -- "Sw3 "/LConn1
  Tap8/RConn1 -- "Sw8 "/LConn1
  Tap7/RConn1 -- "Sw7 "/LConn1
  Tap9/RConn1 -- Sw9/LConn1
  Tap10/RConn1 -- Sw10/LConn1
  Tap11/RConn1 -- Sw11/LConn1
  Tap13/RConn1 -- Sw13/LConn1
  Tap12/RConn1 -- Sw12/LConn1
  Tap14/RConn1 -- Sw14/LConn1
  Tap15/RConn1 -- Sw15/LConn1
  Tap16/RConn1 -- Sw16/LConn1
  Tap17/RConn1 -- Sw17/LConn1
  Tap18/RConn1 -- Sw18/LConn1
  Tap19/RConn1 -- Sw19/LConn1
  Tap20/RConn1 -- Sw20/LConn1

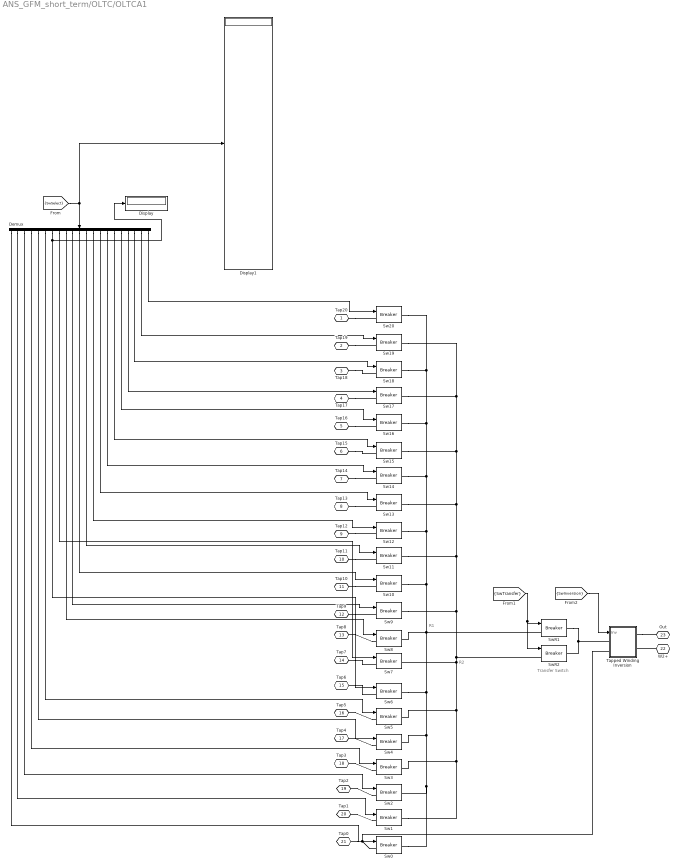
== system ANS_GFM_short_term/OLTC/OLTCA1 ==
  note: R2
  note: R1
  note: Transfer Switch
  Demux : Demux  Outputs=21
      settings: DisplayOption=none
  Display : Display
  Display1 : Display
  "Sw0 " : spsBreakerLib/Breaker  InitialState=InitialStates(1)  SwitchingTimes="[ 1/60  5/60 ]"  External=on  BreakerResistance=Rswitch  SnubberResistance=1e8  SnubberCapacitance=inf  Measurements=None  MoreParameters=off  NoBreakLoop=off
      settings: SourceProductBaseCode=PS
  "Sw1 " : spsBreakerLib/Breaker  InitialState=InitialStates(2)  SwitchingTimes="[ 1/60  5/60 ]"  External=on  BreakerResistance=Rswitch  SnubberResistance=1e8  SnubberCapacitance=inf  Measurements=None  MoreParameters=off  NoBreakLoop=off
      settings: SourceProductBaseCode=PS
  Sw10 : spsBreakerLib/Breaker  InitialState=InitialStates(11)  SwitchingTimes="[ 1/60  5/60 ]"  External=on  BreakerResistance=Rswitch  SnubberResistance=1e8  SnubberCapacitance=inf  Measurements=None  MoreParameters=off  NoBreakLoop=off
      settings: SourceProductBaseCode=PS
  Sw11 : spsBreakerLib/Breaker  InitialState=InitialStates(12)  SwitchingTimes="[ 1/60  5/60 ]"  External=on  BreakerResistance=Rswitch  SnubberResistance=1e8  SnubberCapacitance=inf  Measurements=None  MoreParameters=off  NoBreakLoop=off
      settings: SourceProductBaseCode=PS
  Sw12 : spsBreakerLib/Breaker  InitialState=InitialStates(13)  SwitchingTimes="[ 1/60  5/60 ]"  External=on  BreakerResistance=Rswitch  SnubberResistance=1e8  SnubberCapacitance=inf  Measurements=None  MoreParameters=off  NoBreakLoop=off
      settings: SourceProductBaseCode=PS
  Sw13 : spsBreakerLib/Breaker  InitialState=InitialStates(14)  SwitchingTimes="[ 1/60  5/60 ]"  External=on  BreakerResistance=Rswitch  SnubberResistance=1e8  SnubberCapacitance=inf  Measurements=None  MoreParameters=off  NoBreakLoop=off
      settings: SourceProductBaseCode=PS
  Sw14 : spsBreakerLib/Breaker  InitialState=InitialStates(15)  SwitchingTimes="[ 1/60  5/60 ]"  External=on  BreakerResistance=Rswitch  SnubberResistance=1e8  SnubberCapacitance=inf  Measurements=None  MoreParameters=off  NoBreakLoop=off
      settings: SourceProductBaseCode=PS
  Sw15 : spsBreakerLib/Breaker  InitialState=InitialStates(16)  SwitchingTimes="[ 1/60  5/60 ]"  External=on  BreakerResistance=Rswitch  SnubberResistance=1e8  SnubberCapacitance=inf  Measurements=None  MoreParameters=off  NoBreakLoop=off
      settings: SourceProductBaseCode=PS
  Sw16 : spsBreakerLib/Breaker  InitialState=InitialStates(17)  SwitchingTimes="[ 1/60  5/60 ]"  External=on  BreakerResistance=Rswitch  SnubberResistance=1e8  SnubberCapacitance=inf  Measurements=None  MoreParameters=off  NoBreakLoop=off
      settings: SourceProductBaseCode=PS
  Sw17 : spsBreakerLib/Breaker  InitialState=InitialStates(18)  SwitchingTimes="[ 1/60  5/60 ]"  External=on  BreakerResistance=Rswitch  SnubberResistance=1e8  SnubberCapacitance=inf  Measurements=None  MoreParameters=off  NoBreakLoop=off
      settings: SourceProductBaseCode=PS
  Sw18 : spsBreakerLib/Breaker  InitialState=InitialStates(19)  SwitchingTimes="[ 1/60  5/60 ]"  External=on  BreakerResistance=Rswitch  SnubberResistance=1e8  SnubberCapacitance=inf  Measurements=None  MoreParameters=off  NoBreakLoop=off
      settings: SourceProductBaseCode=PS
  Sw19 : spsBreakerLib/Breaker  InitialState=InitialStates(20)  SwitchingTimes="[ 1/60  5/60 ]"  External=on  BreakerResistance=Rswitch  SnubberResistance=1e8  SnubberCapacitance=inf  Measurements=None  MoreParameters=off  NoBreakLoop=off
      settings: SourceProductBaseCode=PS
  "Sw2 " : spsBreakerLib/Breaker  InitialState=InitialStates(3)  SwitchingTimes="[ 1/60  5/60 ]"  External=on  BreakerResistance=Rswitch  SnubberResistance=1e8  SnubberCapacitance=inf  Measurements=None  MoreParameters=off  NoBreakLoop=off
      settings: SourceProductBaseCode=PS
  Sw20 : spsBreakerLib/Breaker  InitialState=InitialStates(21)  SwitchingTimes="[ 1/60  5/60 ]"  External=on  BreakerResistance=Rswitch  SnubberResistance=Rsnubber  SnubberCapacitance=inf  Measurements=None  MoreParameters=off  NoBreakLoop=off
      settings: SourceProductBaseCode=PS
  "Sw3 " : spsBreakerLib/Breaker  InitialState=InitialStates(4)  SwitchingTimes="[ 1/60  5/60 ]"  External=on  BreakerResistance=Rswitch  SnubberResistance=1e8  SnubberCapacitance=inf  Measurements=None  MoreParameters=off  NoBreakLoop=off
      settings: SourceProductBaseCode=PS
  "Sw4 " : spsBreakerLib/Breaker  InitialState=InitialStates(5)  SwitchingTimes="[ 1/60  5/60 ]"  External=on  BreakerResistance=Rswitch  SnubberResistance=1e8  SnubberCapacitance=inf  Measurements=None  MoreParameters=off  NoBreakLoop=off
      settings: SourceProductBaseCode=PS
  "Sw5 " : spsBreakerLib/Breaker  InitialState=InitialStates(6)  SwitchingTimes="[ 1/60  5/60 ]"  External=on  BreakerResistance=Rswitch  SnubberResistance=1e8  SnubberCapacitance=inf  Measurements=None  MoreParameters=off  NoBreakLoop=off
      settings: SourceProductBaseCode=PS
  "Sw6 " : spsBreakerLib/Breaker  InitialState=InitialStates(7)  SwitchingTimes="[ 1/60  5/60 ]"  External=on  BreakerResistance=Rswitch  SnubberResistance=1e8  SnubberCapacitance=inf  Measurements=None  MoreParameters=off  NoBreakLoop=off
      settings: SourceProductBaseCode=PS
  "Sw7 " : spsBreakerLib/Breaker  InitialState=InitialStates(8)  SwitchingTimes="[ 1/60  5/60 ]"  External=on  BreakerResistance=Rswitch  SnubberResistance=1e8  SnubberCapacitance=inf  Measurements=None  MoreParameters=off  NoBreakLoop=off
      settings: SourceProductBaseCode=PS
  "Sw8 " : spsBreakerLib/Breaker  InitialState=InitialStates(9)  SwitchingTimes="[ 1/60  5/60 ]"  External=on  BreakerResistance=Rswitch  SnubberResistance=1e8  SnubberCapacitance=inf  Measurements=None  MoreParameters=off  NoBreakLoop=off
      settings: SourceProductBaseCode=PS
  Sw9 : spsBreakerLib/Breaker  InitialState=InitialStates(10)  SwitchingTimes="[ 1/60  5/60 ]"  External=on  BreakerResistance=Rswitch  SnubberResistance=1e8  SnubberCapacitance=inf  Measurements=None  MoreParameters=off  NoBreakLoop=off
      settings: SourceProductBaseCode=PS
  SwR1 : spsBreakerLib/Breaker  InitialState=1  SwitchingTimes="[ 1/60  5/60 ]"  External=on  BreakerResistance=Rswitch  SnubberResistance=Rtransfer  SnubberCapacitance=inf  Measurements=None  MoreParameters=off  NoBreakLoop=off
      settings: SourceProductBaseCode=PS
  SwR2 : spsBreakerLib/Breaker  InitialState=1  SwitchingTimes="[ 1/60  5/60 ]"  External=on  BreakerResistance=Rswitch  SnubberResistance=Rtransfer  SnubberCapacitance=inf  Measurements=None  MoreParameters=off  NoBreakLoop=off
      settings: SourceProductBaseCode=PS
  Tapped Winding Inversion : Subsystem
  Tap20 : PMIOPort  Side=Right
  Tap19 : PMIOPort  Port=2  Side=Right
  Tap18 : PMIOPort  Port=3  Side=Right
  Tap17 : PMIOPort  Port=4  Side=Right
  Tap16 : PMIOPort  Port=5  Side=Right
  Tap15 : PMIOPort  Port=6  Side=Right
  Tap14 : PMIOPort  Port=7  Side=Right
  Tap13 : PMIOPort  Port=8  Side=Right
  Tap12 : PMIOPort  Port=9  Side=Right
  Tap11 : PMIOPort  Port=10  Side=Right
  Tap10 : PMIOPort  Port=11  Side=Right
  Tap9 : PMIOPort  Port=12  Side=Right
  Tap8 : PMIOPort  Port=13  Side=Right
  Tap7 : PMIOPort  Port=14  Side=Right
  Tap6 : PMIOPort  Port=15  Side=Right
  Tap5 : PMIOPort  Port=16  Side=Right
  Tap4 : PMIOPort  Port=17  Side=Right
  Tap3 : PMIOPort  Port=18  Side=Right
  Tap2 : PMIOPort  Port=19  Side=Right
  Tap1 : PMIOPort  Port=20  Side=Right
  Tap0 : PMIOPort  Port=21  Side=Right
  W2+ : PMIOPort  Port=22  Side=Right
  Out : PMIOPort  Port=23  Side=Left
  wires:
  Demux/9 -> "Sw8 "/1
  Demux/8 -> "Sw7 "/1
  Demux/7 -> Display/1, "Sw6 "/1
  Demux/6 -> "Sw5 "/1
  Demux/5 -> "Sw4 "/1
  Demux/4 -> "Sw3 "/1
  Demux/3 -> "Sw2 "/1
  Demux/2 -> "Sw1 "/1
  Demux/1 -> "Sw0 "/1
  [SwInversion] -> Tapped Winding Inversion/1(Inv)
  [SwTransfer] -> SwR2/1, SwR1/1
  [SwSelect] -> Demux/1, Display1/1
  Demux/10 -> Sw9/1
  Demux/11 -> Sw10/1
  Demux/12 -> Sw11/1
  Demux/13 -> Sw12/1
  Demux/14 -> Sw13/1
  Demux/15 -> Sw14/1
  Demux/16 -> Sw15/1
  Demux/17 -> Sw16/1
  Demux/18 -> Sw17/1
  Demux/19 -> Sw18/1
  Demux/20 -> Sw19/1
  Demux/21 -> Sw20/1
  connections:
  "Sw0 "/LConn1 -- Tap0/RConn1 -- Tapped Winding Inversion/LConn2
  Tap1/RConn1 -- "Sw1 "/LConn1
  Tap2/RConn1 -- "Sw2 "/LConn1
  Tap6/RConn1 -- "Sw6 "/LConn1
  Tap4/RConn1 -- "Sw4 "/LConn1
  Tap5/RConn1 -- "Sw5 "/LConn1
  SwR1/RConn1 -- Tapped Winding Inversion/LConn1 -- SwR2/RConn1
  Sw19/RConn1 -- Sw17/RConn1 -- Sw15/RConn1 -- Sw13/RConn1 -- Sw11/RConn1 -- Sw9/RConn1 -- SwR2/LConn1 -- "Sw5 "/RConn1 -- "Sw3 "/RConn1 -- "Sw1 "/RConn1 -- "Sw7 "/RConn1
  Tapped Winding Inversion/RConn1 -- Out/RConn1
  W2+/RConn1 -- Tapped Winding Inversion/RConn2
  "Sw6 "/RConn1 -- "Sw4 "/RConn1 -- "Sw2 "/RConn1 -- "Sw0 "/RConn1 -- Sw20/RConn1 -- Sw18/RConn1 -- Sw16/RConn1 -- Sw14/RConn1 -- Sw12/RConn1 -- Sw10/RConn1 -- "Sw8 "/RConn1 -- SwR1/LConn1
  Tap3/RConn1 -- "Sw3 "/LConn1
  Tap8/RConn1 -- "Sw8 "/LConn1
  Tap7/RConn1 -- "Sw7 "/LConn1
  Tap9/RConn1 -- Sw9/LConn1
  Tap10/RConn1 -- Sw10/LConn1
  Tap11/RConn1 -- Sw11/LConn1
  Tap13/RConn1 -- Sw13/LConn1
  Tap12/RConn1 -- Sw12/LConn1
  Tap14/RConn1 -- Sw14/LConn1
  Tap15/RConn1 -- Sw15/LConn1
  Tap16/RConn1 -- Sw16/LConn1
  Tap17/RConn1 -- Sw17/LConn1
  Tap18/RConn1 -- Sw18/LConn1
  Tap19/RConn1 -- Sw19/LConn1
  Tap20/RConn1 -- Sw20/LConn1
